simulink model "aircraft_model_2014"  (R2014a)
settings: Solver=ode45  SolverMode=SingleTasking  StartTime=0.0  StopTime=150  RelTol=1e-3
values from neighbouring files (symbols this model uses):
  g = 9.8    [model.mat]
  Kd = 1e-06    [model.mat]
  Kt = 1    [model.mat]
  U0 = 120    [model.mat]
  X0 = 0    [model.mat]
  Y0 = 5000    [model.mat]
undefined symbols (not defined in the file or in its folder): magnitude
libraries: simulink x1
settings Model: CovMetricSettings=dwe  CovHtmlReporting=off  covSaveCumulativeToWorkspaceVar=off  CovSaveSingleToWorkspaceVar=off  CovExternalEMLEnable=on  CovSFcnEnable=on  Creator=jomig  LastModifiedBy=jomig
settings DataIOCC: LimitDataPoints=off  SaveFormat=StructureWithTime
settings DebuggingCC: MergeDetectMultiDrivingBlocksExec=error  SolverPrmCheckMsg=none  FrameProcessingCompatibilityMsg=error  SFUnexpectedBacktrackingDiag=error  SFNoUnconditionalDefaultTransitionDiag=error
settings HardwareCC: ProdBitPerPointer=64  ProdLargestAtomicFloat=Float  ProdIntDivRoundTo=Zero  ProdEndianess=LittleEndian  ProdHWDeviceType=Specified
settings ModelReferenceCC: PropagateSignalLabelsOutOfModel=on
settings GRTTargetCC: TargetLangStandard=C99 (ISO)  GeneratePreprocessorConditionals=Use local settings

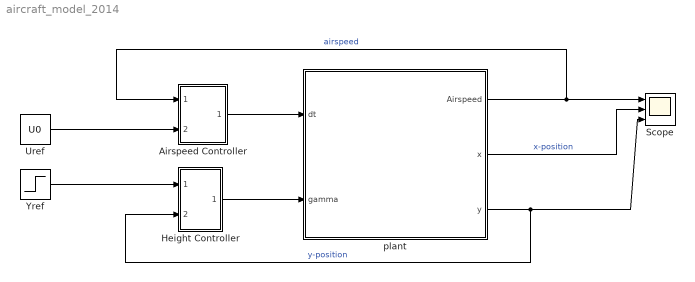
== system aircraft_model_2014 ==
  Airspeed Controller : Subsystem
  Height Controller : Subsystem
  Scope : Scope  NumInputPorts=3
      settings: TimeRange=auto  MaxDataPoints=5000  SaveToWorkspace=off  SaveName=ScopeData  YMin=119.68678~-2248.45799~4937.50109  YMax=120.36014~20236.12191~5562.49019  SampleTime=-1
  "Uref " : Constant  Value=U0
  Yref : Step  Time=5  Before=Y0  After=Y0+500  SampleTime=0
  "plant " : Subsystem
  wires:
  "plant "/2(x) -> Scope/2  "x-position"
  "plant "/3(y) -> Height Controller/2(y_hat), Scope/3  "y-position"
  "plant "/1(Airspeed) -> Scope/1, Airspeed Controller/1(U_hat)  "airspeed"
  "Uref "/1 -> Airspeed Controller/2(U_ref)
  Airspeed Controller/1(Throtle) -> "plant "/1(dt)
  Yref/1 -> Height Controller/1(y_ref)
  Height Controller/1(gamma) -> "plant "/2("gamma ")

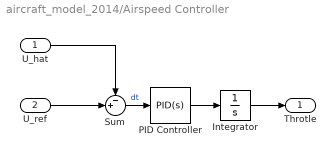
== system aircraft_model_2014/Airspeed Controller ==
  U_hat : Inport
  U_ref : Inport  Port=2
  Integrator : Integrator
  PID Controller : simulink/Continuous/PID Controller  Controller=PID  TimeDomain=Continuous-time  SampleTime=-1  IntegratorMethod=Forward Euler  FilterMethod=Forward Euler  Form=Parallel  UseFilter=on  ControllerParametersSource=internal  P=0.3  I=0.215  D=1.1625  N=100  InitialConditionSource=internal  InitialConditionForIntegrator=0  InitialConditionForFilter=0  ExternalReset=none  LimitOutput=off  UpperSaturationLimit=inf  LowerSaturationLimit=-inf  LinearizeAsGain=on  AntiWindupMode=none  Kb=1  TrackingMode=off  Kt=1  PParamMin=[]  PParamMax=[]  IParamMin=[]  IParamMax=[]  DParamMin=[]  DParamMax=[]  NParamMin=[]  NParamMax=[]  KbParamMin=[]  KbParamMax=[]  KtParamMin=[]  KtParamMax=[]  POutMin=[]  POutMax=[]  IOutMin=[]  IOutMax=[]  DOutMin=[]  DOutMax=[]  NOutMin=[]  NOutMax=[]  KbOutMin=[]  KbOutMax=[]  KtOutMin=[]  KtOutMax=[]  IntegratorOutMin=[]  IntegratorOutMax=[]  FilterOutMin=[]  FilterOutMax=[]  SumOutMin=[]  SumOutMax=[]  SumI1OutMin=[]  SumI1OutMax=[]  SumI2OutMin=[]  SumI2OutMax=[]  SumI3OutMin=[]  SumI3OutMax=[]  SumDOutMin=[]  SumDOutMax=[]  SaturationOutMin=[]  SaturationOutMax=[]  IntegratorContinuousStateAttributes=''  IntegratorStateMustResolveToSignalObject=off  IntegratorRTWStateStorageClass=Auto  FilterContinuousStateAttributes=''  FilterStateMustResolveToSignalObject=off  FilterRTWStateStorageClass=Auto  DifferentiatorICPrevScaledInput=0  DifferentiatorOutMin=[]  DifferentiatorOutMax=[]
  Sum : Sum  Inputs=-+|
  Throtle : Outport
  wires:
  PID Controller/1 -> Integrator/1
  U_ref/1 -> Sum/2
  Integrator/1 -> Throtle/1
  U_hat/1 -> Sum/1
  Sum/1 -> PID Controller/1  "dt"

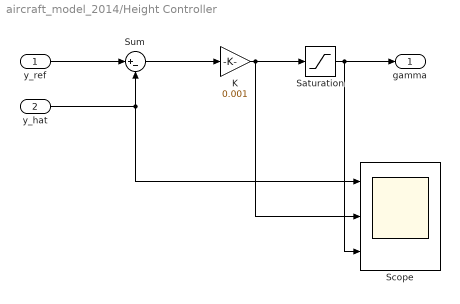
== system aircraft_model_2014/Height Controller ==
  y_ref : Inport
  y_hat : Inport  Port=2
  K : Gain  Gain=0.001
  Saturation : Saturate  UpperLimit=3*pi/180  LowerLimit=-3*pi/180
  Scope : Scope  NumInputPorts=3
      settings: TimeRange=auto  MaxDataPoints=5000  SaveToWorkspace=off  SaveName=ScopeData2  YMin=4937.50109~-0.0625~-0.00654  YMax=5562.49019~0.5625~0.0589  SampleTime=-1
  Sum : Sum  Inputs=|+-
  gamma : Outport
  wires:
  Saturation/1 -> Scope/3, gamma/1
  y_ref/1 -> Sum/1
  y_hat/1 -> Scope/1, Sum/2
  K/1 -> Scope/2, Saturation/1
  Sum/1 -> K/1

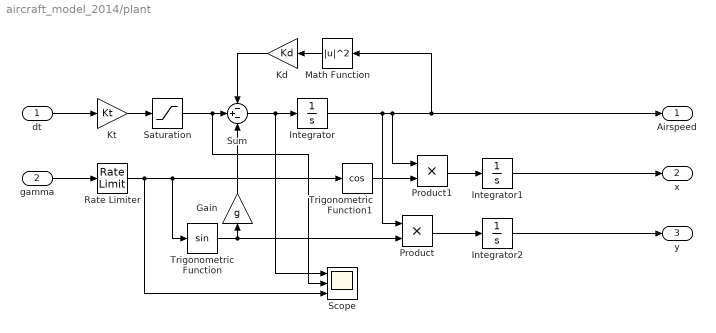
== system aircraft_model_2014/plant  ==
  dt : Inport
  "gamma " : Inport  Port=2
  Gain : Gain  Gain=g
  Integrator : Integrator  InitialCondition=U0
  Integrator1 : Integrator  InitialCondition=X0
  Integrator2 : Integrator  InitialCondition=Y0
  Kd : Gain  Gain=Kd
  Kt : Gain  Gain=Kt
  Math Function : Math  Operator=magnitude^2  SaturateOnIntegerOverflow=on
  Product : Product
  Product1 : Product
  Rate Limiter : RateLimiter  RisingSlewLimit=pi/180  FallingSlewLimit=-pi/180  SampleTimeMode=inherited
  Saturation : Saturate  UpperLimit=15  LowerLimit=0
  Scope : Scope  NumInputPorts=3
      settings: TimeRange=auto  MaxDataPoints=5000  SaveToWorkspace=off  YMin=-0.08421~-0.06411~-0.00654  YMax=0.7579~0.577~0.0589  SampleTime=-1
  Sum : Sum  Inputs=-+-
  Trigonometric Function : Trigonometry
  Trigonometric Function1 : Trigonometry  Operator=cos
  Airspeed : Outport
  x : Outport  Port=2
  y : Outport  Port=3
  wires:
  dt/1 -> Kt/1
  Integrator/1 -> Product/1, Math Function/1, Airspeed/1, Product1/1
  Product/1 -> Integrator2/1
  "gamma "/1 -> Rate Limiter/1
  Integrator1/1 -> x/1
  Trigonometric Function1/1 -> Product1/2
  Product1/1 -> Integrator1/1
  Trigonometric Function/1 -> Gain/1, Product/2
  Integrator2/1 -> y/1
  Sum/1 -> Scope/1, Integrator/1
  Kt/1 -> Saturation/1
  Kd/1 -> Sum/1
  Math Function/1 -> Kd/1
  Gain/1 -> Sum/3
  Rate Limiter/1 -> Scope/3, Trigonometric Function1/1, Trigonometric Function/1
  Saturation/1 -> Scope/2, Sum/2
